simulink model "Simulink_Parctica_1"  (R2024b)
settings: Solver=VariableStepAuto  StartTime=0.0  StopTime=10.0  RelTol=1e-3
values from neighbouring files (symbols this model uses):
  A = (Ip + (Mp * Lp^2)) * Beq    (= 0.14180268756)    [Practica_1.m]
  alpha0 = deg2rad(1)    [Practica_1.m]
  B = (Mp^2) * (Lp^2) * g    (= 0.056582068126)    [Practica_1.m]
  C = (Ip * Mp * Lp) - ((Mp^2) * (Lp^3))    (= -0.00130455248126)    [Practica_1.m]
  D = Mp * Lp * Bp    (= 0.0001822704)    [Practica_1.m]
  Den = (M * Ip) + (Mc * Mp * (Lp^2))    (= 0.0250033882845)    [Practica_1.m]
  E = M * Mp * Lp * g    (= 0.695187735606)    [Practica_1.m]
  F = M * Bp    (= 0.00223944)    [Practica_1.m]
  G = Mp^2 * Lp^2    (= 0.005767794916)    [Practica_1.m]
  H = Beq * Mp * Lp    (= 0.3265678)    [Practica_1.m]
  I = (Mp^2) * (Lp^2)    (= 0.005767794916)    [Practica_1.m]
settings Model: Creator=mac09  LastModifiedBy=mac09

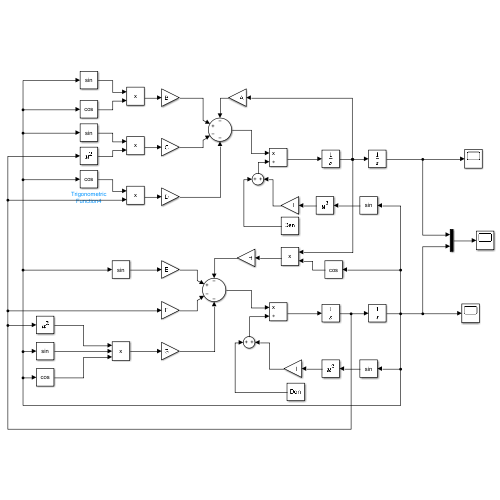
[thumbnail: Simulink's stored preview of the top-level diagram]
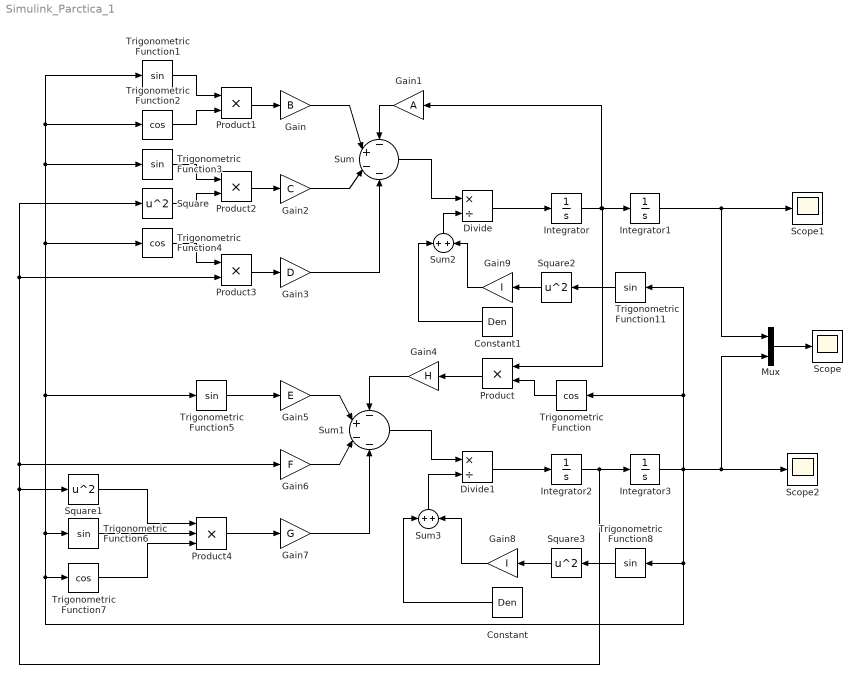
== system Simulink_Parctica_1 ==
  Constant : Constant  Value=Den
  Constant1 : Constant  Value=Den
  Divide : Product  Inputs=*/
  Divide1 : Product  Inputs=*/
  Gain : Gain  Gain=B
  Gain1 : Gain  Gain=A
  Gain2 : Gain  Gain=C
  Gain3 : Gain  Gain=D
  Gain4 : Gain  Gain=H
  Gain5 : Gain  Gain=E
  Gain6 : Gain  Gain=F
  Gain7 : Gain  Gain=G
  Gain8 : Gain  Gain=I
  Gain9 : Gain  Gain=I
  Integrator : Integrator
  Integrator1 : Integrator
  Integrator2 : Integrator
  Integrator3 : Integrator  InitialCondition=alpha0
  Mux : Mux  Inputs=2
  Product{,1..3} (4 alike) : Product
  Product4 : Product  Inputs=3
  Scope : Scope
  Scope1 : Scope
  Scope2 : Scope
  Square{,1..3} (4 alike) : Math  Operator=square
  Sum : Sum  Inputs=-|+|-|-
  Sum1 : Sum  Inputs=-|+|-|-
  Sum2 : Sum  Inputs=+|+
  Sum3 : Sum  Inputs=+|+
  Trigonometric Function{,2,4,7} (4 alike) : Trigonometry  Operator=cos
  Trigonometric Function{1,3,5..6,8,11} (6 alike) : Trigonometry
  wires:
  Divide/1 -> Integrator/1
  Integrator2/1 -> Square/1, Product3/2, Gain6/1, Square1/1, Integrator3/1
  Divide1/1 -> Integrator2/1
  Sum/1 -> Divide/1
  Sum1/1 -> Divide1/1
  Gain/1 -> Sum/2
  Gain1/1 -> Sum/1
  Integrator/1 -> Gain1/1, Product/1, Integrator1/1
  Gain2/1 -> Sum/3
  Gain3/1 -> Sum/4
  Gain4/1 -> Sum1/1
  Trigonometric Function/1 -> Product/2
  Integrator3/1 -> Trigonometric Function11/1, Trigonometric Function/1, Scope2/1, Mux/2, Trigonometric Function8/1, Trigonometric Function7/1, Trigonometric Function6/1, Trigonometric Function5/1, Trigonometric Function1/1, Trigonometric Function2/1, Trigonometric Function3/1, Trigonometric Function4/1
  Product/1 -> Gain4/1
  Gain5/1 -> Sum1/2
  Gain6/1 -> Sum1/3
  Gain7/1 -> Sum1/4
  Product1/1 -> Gain/1
  Trigonometric Function1/1 -> Product1/1
  Trigonometric Function2/1 -> Product1/2
  Product2/1 -> Gain2/1
  Trigonometric Function3/1 -> Product2/1
  Square/1 -> Product2/2
  Product3/1 -> Gain3/1
  Trigonometric Function4/1 -> Product3/1
  Trigonometric Function5/1 -> Gain5/1
  Product4/1 -> Gain7/1
  Trigonometric Function6/1 -> Product4/2
  Trigonometric Function7/1 -> Product4/3
  Square1/1 -> Product4/1
  Sum3/1 -> Divide1/2
  Square3/1 -> Gain8/1
  Gain8/1 -> Sum3/2
  Sum2/1 -> Divide/2
  Trigonometric Function11/1 -> Square2/1
  Square2/1 -> Gain9/1
  Gain9/1 -> Sum2/2
  Constant1/1 -> Sum2/1
  Integrator1/1 -> Mux/1, Scope1/1
  Mux/1 -> Scope/1
  Constant/1 -> Sum3/1
  Trigonometric Function8/1 -> Square3/1
